simulink model "MVB1 - 副本"  (R2013b)
settings: Solver=ode3  StartTime=0.0  StopTime=6e-5  RelTol=1e-3
libraries: simulink x4
settings Model: Creator=qiji  LastModifiedBy=qiji
settings DataIOCC: SignalLoggingSaveFormat=ModelDataLogs
settings DebuggingCC: UnderspecifiedInitializationDetection=Simplified  MultiTaskDSMMsg=warning  MultiTaskCondExecSysMsg=none  SFUnusedDataAndEventsDiag=none
settings RTWCC: IncludeERTFirstTime=on
settings GRTTargetCC: CodeReplacementLibrary=None  CPPClassGenCompliant=on

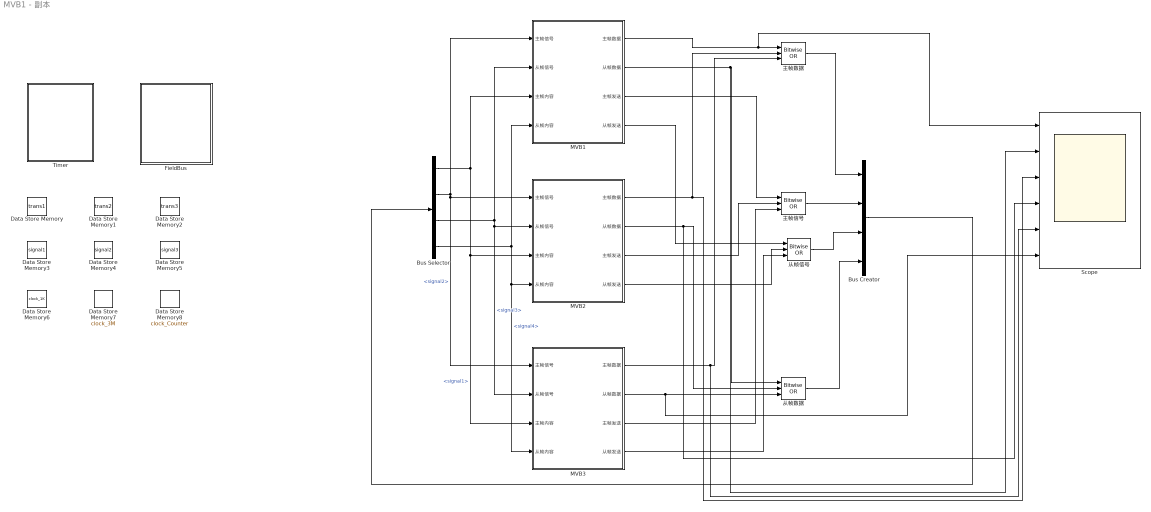
== system MVB1 - 副本 ==
  Bus Creator : BusCreator
  Bus Selector : BusSelector  OutputSignals=signal1,signal2,signal3,signal4
  Data Store Memory : DataStoreMemory  DataStoreName=trans1  ReadBeforeWriteMsg=warning  WriteAfterWriteMsg=warning  WriteAfterReadMsg=warning  OutDataTypeStr=boolean
  Data Store Memory1 : DataStoreMemory  DataStoreName=trans2  ReadBeforeWriteMsg=warning  WriteAfterWriteMsg=warning  WriteAfterReadMsg=warning  OutDataTypeStr=boolean
  Data Store Memory2 : DataStoreMemory  DataStoreName=trans3  ReadBeforeWriteMsg=warning  WriteAfterWriteMsg=warning  WriteAfterReadMsg=warning  OutDataTypeStr=boolean
  Data Store Memory3 : DataStoreMemory  DataStoreName=signal1  ReadBeforeWriteMsg=warning  WriteAfterWriteMsg=warning  WriteAfterReadMsg=warning  OutDataTypeStr=boolean
  Data Store Memory4 : DataStoreMemory  DataStoreName=signal2  ReadBeforeWriteMsg=warning  WriteAfterWriteMsg=warning  WriteAfterReadMsg=warning  OutDataTypeStr=boolean
  Data Store Memory5 : DataStoreMemory  DataStoreName=signal3  ReadBeforeWriteMsg=warning  WriteAfterWriteMsg=warning  WriteAfterReadMsg=warning  OutDataTypeStr=boolean
  Data Store Memory6 : DataStoreMemory  DataStoreName=clock_1K  ReadBeforeWriteMsg=warning  WriteAfterWriteMsg=warning  WriteAfterReadMsg=warning  OutDataTypeStr=boolean
  Data Store Memory7 : DataStoreMemory  DataStoreName=clock_3M  ReadBeforeWriteMsg=warning  WriteAfterWriteMsg=warning  WriteAfterReadMsg=warning  OutDataTypeStr=boolean
  Data Store Memory8 : DataStoreMemory  DataStoreName=clock_Counter  ReadBeforeWriteMsg=warning  WriteAfterWriteMsg=warning  WriteAfterReadMsg=warning  OutDataTypeStr=uint32
  FieldBus : Subsystem
  MVB1 : Subsystem
  MVB2 : Subsystem
  MVB3 : Subsystem
  Scope : Scope  NumInputPorts=6
      settings: YMin=0~0~0~0~0~0  YMax=3.5e+09~3e+09~3.5e+09~3e+09~3.5e+09~3e+09
  Timer : Subsystem
  主帧信号 : simulink/Logic and Bit Operations/Bitwise Operator  logicop=OR  UseBitMask=off  NumInputPorts=3  BitMask=bin2dec('11011001')  BitMaskRealWorld=Stored Integer
  主帧数据 : simulink/Logic and Bit Operations/Bitwise Operator  logicop=OR  UseBitMask=off  NumInputPorts=3  BitMask=bin2dec('11011001')  BitMaskRealWorld=Stored Integer
  从帧信号 : simulink/Logic and Bit Operations/Bitwise Operator  logicop=OR  UseBitMask=off  NumInputPorts=3  BitMask=bin2dec('11011001')  BitMaskRealWorld=Stored Integer
  从帧数据 : simulink/Logic and Bit Operations/Bitwise Operator  logicop=OR  UseBitMask=off  NumInputPorts=3  BitMask=bin2dec('11011001')  BitMaskRealWorld=Stored Integer
  wires:
  MVB1/1(主帧数据) -> Scope/1, 主帧数据/1
  MVB2/1(主帧数据) -> Scope/3, 主帧数据/2
  MVB3/1(主帧数据) -> Scope/5, 主帧数据/3
  MVB1/2(从帧数据) -> Scope/2, 从帧数据/1
  MVB2/2(从帧数据) -> 从帧数据/2, Scope/4
  MVB3/2(从帧数据) -> Scope/6, 从帧数据/3
  MVB1/3(主帧发送) -> 主帧信号/1
  MVB2/3(主帧发送) -> 主帧信号/2
  MVB3/3(主帧发送) -> 主帧信号/3
  MVB1/4(从帧发送) -> 从帧信号/1
  MVB2/4(从帧发送) -> 从帧信号/2
  MVB3/4(从帧发送) -> 从帧信号/3
  主帧数据/1 -> Bus Creator/1
  主帧信号/1 -> Bus Creator/2
  从帧信号/1 -> Bus Creator/3
  从帧数据/1 -> Bus Creator/4
  Bus Creator/1 -> Bus Selector/1
  Bus Selector/1 -> MVB2/3(主帧内容), MVB3/3(主帧内容), MVB1/3(主帧内容)  "<signal1>"
  Bus Selector/2 -> MVB3/1(主帧信号), MVB2/1(主帧信号), MVB1/1(主帧信号)  "<signal2>"
  Bus Selector/3 -> MVB3/2(从帧信号), MVB2/2(从帧信号), MVB1/2(从帧信号)  "<signal3>"
  Bus Selector/4 -> MVB3/4(从帧内容), MVB2/4(从帧内容), MVB1/4(从帧内容)  "<signal4>"

== system MVB1 - 副本/FieldBus ==
  FIELDBUS : Stateflow chart  TreatAsAtomicUnit=on

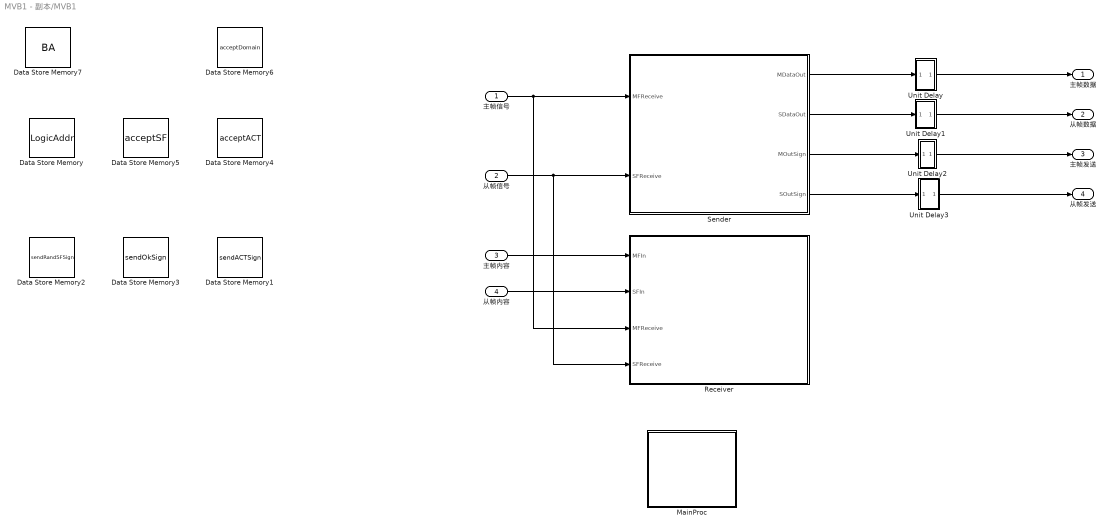
== system MVB1 - 副本/MVB1 ==
  主帧信号 : Inport
  从帧信号 : Inport  Port=2
  主帧内容 : Inport  Port=3
  从帧内容 : Inport  Port=4
  Data Store Memory : DataStoreMemory  DataStoreName=LogicAddr  ReadBeforeWriteMsg=warning  WriteAfterWriteMsg=warning  WriteAfterReadMsg=warning  InitialValue=1  OutDataTypeStr=uint32
  Data Store Memory1 : DataStoreMemory  DataStoreName=sendACTSign  ReadBeforeWriteMsg=warning  WriteAfterWriteMsg=warning  WriteAfterReadMsg=warning  OutDataTypeStr=boolean
  Data Store Memory2 : DataStoreMemory  DataStoreName=sendRandSFSign  ReadBeforeWriteMsg=warning  WriteAfterWriteMsg=warning  WriteAfterReadMsg=warning  OutDataTypeStr=boolean
  Data Store Memory3 : DataStoreMemory  DataStoreName=sendOkSign  ReadBeforeWriteMsg=warning  WriteAfterWriteMsg=warning  WriteAfterReadMsg=warning  OutDataTypeStr=boolean
  Data Store Memory4 : DataStoreMemory  DataStoreName=acceptACT  ReadBeforeWriteMsg=warning  WriteAfterWriteMsg=warning  WriteAfterReadMsg=warning  InitialValue=false  OutDataTypeStr=boolean
  Data Store Memory5 : DataStoreMemory  DataStoreName=acceptSF  ReadBeforeWriteMsg=warning  WriteAfterWriteMsg=warning  WriteAfterReadMsg=warning  InitialValue=false  OutDataTypeStr=boolean
  Data Store Memory6 : DataStoreMemory  DataStoreName=acceptDomain  ReadBeforeWriteMsg=warning  WriteAfterWriteMsg=warning  WriteAfterReadMsg=warning  InitialValue=false  OutDataTypeStr=boolean
  Data Store Memory7 : DataStoreMemory  DataStoreName=BA  ReadBeforeWriteMsg=warning  WriteAfterWriteMsg=warning  WriteAfterReadMsg=warning  InitialValue=true  OutDataTypeStr=boolean
  MainProc : Stateflow chart  TreatAsAtomicUnit=on
  Receiver : Stateflow chart  TreatAsAtomicUnit=on
  Sender : Stateflow chart  TreatAsAtomicUnit=on
  Unit Delay : Subsystem
  Unit Delay1 : Subsystem
  Unit Delay2 : Subsystem
  Unit Delay3 : Subsystem
  主帧数据 : Outport
  从帧数据 : Outport  Port=2
  主帧发送 : Outport  Port=3
  从帧发送 : Outport  Port=4
  wires:
  Sender/1(MDataOut) -> Unit Delay/1(In1)
  Sender/2(SDataOut) -> Unit Delay1/1(In1)
  Sender/3(MOutSign) -> Unit Delay2/1(In1)
  Sender/4(SOutSign) -> Unit Delay3/1(In1)
  Unit Delay/1(Out1) -> 主帧数据/1
  Unit Delay1/1(Out1) -> 从帧数据/1
  Unit Delay2/1(Out1) -> 主帧发送/1
  Unit Delay3/1(Out1) -> 从帧发送/1
  主帧信号/1 -> Receiver/3(MFReceive), Sender/1(MFReceive)
  从帧信号/1 -> Receiver/4(SFReceive), Sender/2(SFReceive)
  主帧内容/1 -> Receiver/1(MFIn)
  从帧内容/1 -> Receiver/2(SFIn)

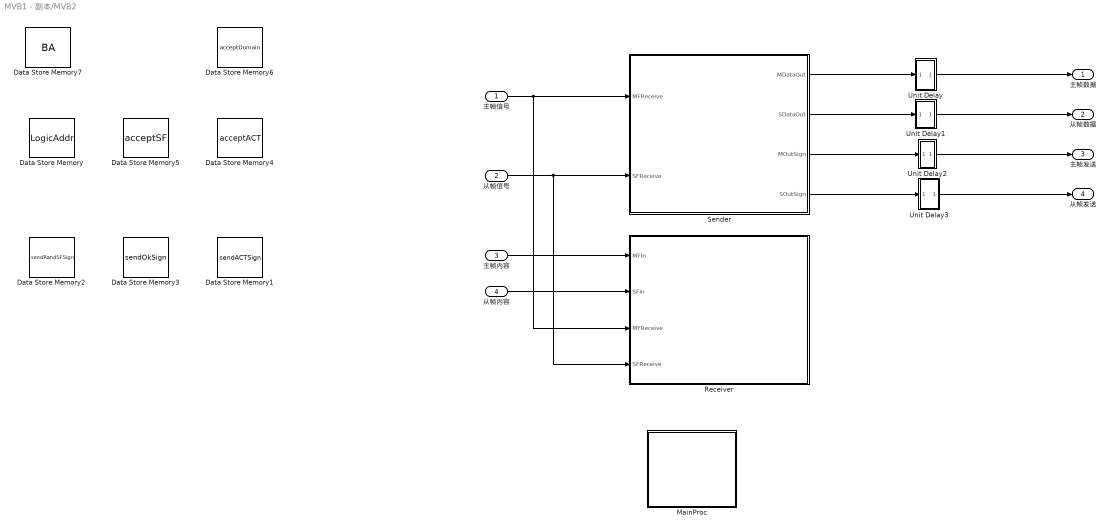
== system MVB1 - 副本/MVB2 ==
  主帧信号 : Inport
  从帧信号 : Inport  Port=2
  主帧内容 : Inport  Port=3
  从帧内容 : Inport  Port=4
  Data Store Memory : DataStoreMemory  DataStoreName=LogicAddr  ReadBeforeWriteMsg=warning  WriteAfterWriteMsg=warning  WriteAfterReadMsg=warning  InitialValue=2  OutDataTypeStr=uint32
  Data Store Memory1 : DataStoreMemory  DataStoreName=sendACTSign  ReadBeforeWriteMsg=warning  WriteAfterWriteMsg=warning  WriteAfterReadMsg=warning  OutDataTypeStr=boolean
  Data Store Memory2 : DataStoreMemory  DataStoreName=sendRandSFSign  ReadBeforeWriteMsg=warning  WriteAfterWriteMsg=warning  WriteAfterReadMsg=warning  OutDataTypeStr=boolean
  Data Store Memory3 : DataStoreMemory  DataStoreName=sendOkSign  ReadBeforeWriteMsg=warning  WriteAfterWriteMsg=warning  WriteAfterReadMsg=warning  OutDataTypeStr=boolean
  Data Store Memory4 : DataStoreMemory  DataStoreName=acceptACT  ReadBeforeWriteMsg=warning  WriteAfterWriteMsg=warning  WriteAfterReadMsg=warning  InitialValue=false  OutDataTypeStr=boolean
  Data Store Memory5 : DataStoreMemory  DataStoreName=acceptSF  ReadBeforeWriteMsg=warning  WriteAfterWriteMsg=warning  WriteAfterReadMsg=warning  InitialValue=false  OutDataTypeStr=boolean
  Data Store Memory6 : DataStoreMemory  DataStoreName=acceptDomain  ReadBeforeWriteMsg=warning  WriteAfterWriteMsg=warning  WriteAfterReadMsg=warning  InitialValue=false  OutDataTypeStr=boolean
  Data Store Memory7 : DataStoreMemory  DataStoreName=BA  ReadBeforeWriteMsg=warning  WriteAfterWriteMsg=warning  WriteAfterReadMsg=warning  InitialValue=true  OutDataTypeStr=boolean
  MainProc : Stateflow chart  TreatAsAtomicUnit=on
  Receiver : Stateflow chart  TreatAsAtomicUnit=on
  Sender : Stateflow chart  TreatAsAtomicUnit=on
  Unit Delay : Subsystem
  Unit Delay1 : Subsystem
  Unit Delay2 : Subsystem
  Unit Delay3 : Subsystem
  主帧数据 : Outport
  从帧数据 : Outport  Port=2
  主帧发送 : Outport  Port=3
  从帧发送 : Outport  Port=4
  wires:
  从帧内容/1 -> Receiver/2(SFIn)
  主帧内容/1 -> Receiver/1(MFIn)
  从帧信号/1 -> Sender/2(SFReceive), Receiver/4(SFReceive)
  主帧信号/1 -> Sender/1(MFReceive), Receiver/3(MFReceive)
  Unit Delay3/1(Out1) -> 从帧发送/1
  Unit Delay2/1(Out1) -> 主帧发送/1
  Unit Delay1/1(Out1) -> 从帧数据/1
  Unit Delay/1(Out1) -> 主帧数据/1
  Sender/4(SOutSign) -> Unit Delay3/1(In1)
  Sender/3(MOutSign) -> Unit Delay2/1(In1)
  Sender/2(SDataOut) -> Unit Delay1/1(In1)
  Sender/1(MDataOut) -> Unit Delay/1(In1)

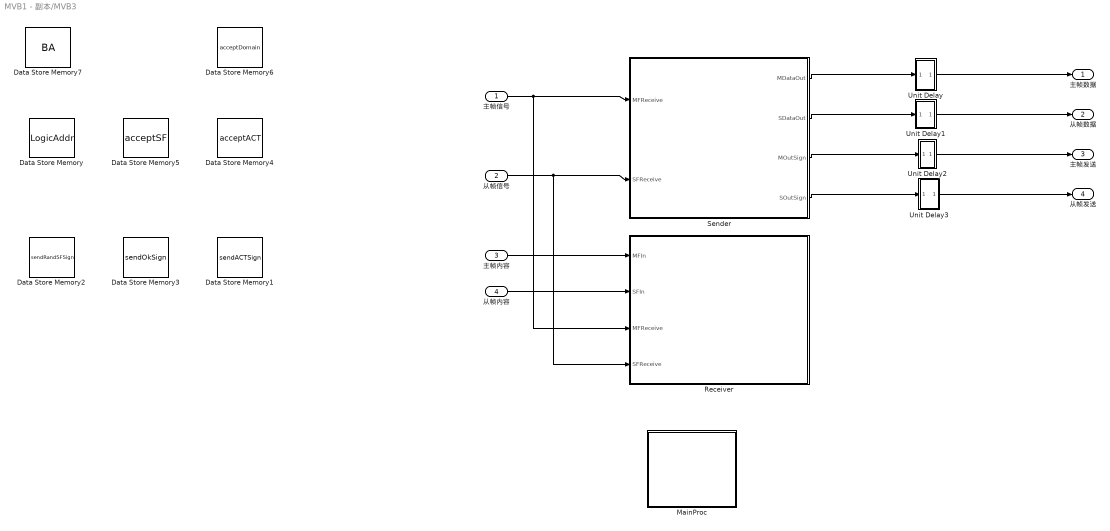
== system MVB1 - 副本/MVB3 ==
  主帧信号 : Inport
  从帧信号 : Inport  Port=2
  主帧内容 : Inport  Port=3
  从帧内容 : Inport  Port=4
  Data Store Memory : DataStoreMemory  DataStoreName=LogicAddr  ReadBeforeWriteMsg=warning  WriteAfterWriteMsg=warning  WriteAfterReadMsg=warning  InitialValue=3  OutDataTypeStr=uint32
  Data Store Memory1 : DataStoreMemory  DataStoreName=sendACTSign  ReadBeforeWriteMsg=warning  WriteAfterWriteMsg=warning  WriteAfterReadMsg=warning  OutDataTypeStr=boolean
  Data Store Memory2 : DataStoreMemory  DataStoreName=sendRandSFSign  ReadBeforeWriteMsg=warning  WriteAfterWriteMsg=warning  WriteAfterReadMsg=warning  OutDataTypeStr=boolean
  Data Store Memory3 : DataStoreMemory  DataStoreName=sendOkSign  ReadBeforeWriteMsg=warning  WriteAfterWriteMsg=warning  WriteAfterReadMsg=warning  OutDataTypeStr=boolean
  Data Store Memory4 : DataStoreMemory  DataStoreName=acceptACT  ReadBeforeWriteMsg=warning  WriteAfterWriteMsg=warning  WriteAfterReadMsg=warning  InitialValue=false  OutDataTypeStr=boolean
  Data Store Memory5 : DataStoreMemory  DataStoreName=acceptSF  ReadBeforeWriteMsg=warning  WriteAfterWriteMsg=warning  WriteAfterReadMsg=warning  InitialValue=false  OutDataTypeStr=boolean
  Data Store Memory6 : DataStoreMemory  DataStoreName=acceptDomain  ReadBeforeWriteMsg=warning  WriteAfterWriteMsg=warning  WriteAfterReadMsg=warning  InitialValue=false  OutDataTypeStr=boolean
  Data Store Memory7 : DataStoreMemory  DataStoreName=BA  ReadBeforeWriteMsg=warning  WriteAfterWriteMsg=warning  WriteAfterReadMsg=warning  InitialValue=true  OutDataTypeStr=boolean
  MainProc : Stateflow chart  TreatAsAtomicUnit=on
  Receiver : Stateflow chart  TreatAsAtomicUnit=on
  Sender : Stateflow chart  TreatAsAtomicUnit=on
  Unit Delay : Subsystem
  Unit Delay1 : Subsystem
  Unit Delay2 : Subsystem
  Unit Delay3 : Subsystem
  主帧数据 : Outport
  从帧数据 : Outport  Port=2
  主帧发送 : Outport  Port=3
  从帧发送 : Outport  Port=4
  wires:
  Sender/1(MDataOut) -> Unit Delay/1(In1)
  Sender/2(SDataOut) -> Unit Delay1/1(In1)
  Sender/3(MOutSign) -> Unit Delay2/1(In1)
  Sender/4(SOutSign) -> Unit Delay3/1(In1)
  Unit Delay/1(Out1) -> 主帧数据/1
  Unit Delay1/1(Out1) -> 从帧数据/1
  Unit Delay2/1(Out1) -> 主帧发送/1
  Unit Delay3/1(Out1) -> 从帧发送/1
  主帧信号/1 -> Receiver/3(MFReceive), Sender/1(MFReceive)
  从帧信号/1 -> Receiver/4(SFReceive), Sender/2(SFReceive)
  主帧内容/1 -> Receiver/1(MFIn)
  从帧内容/1 -> Receiver/2(SFIn)

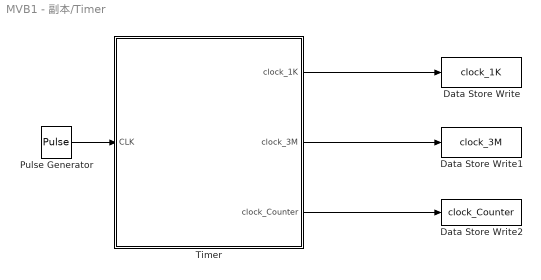
== system MVB1 - 副本/Timer ==
  Data Store Write : DataStoreWrite  DataStoreName=clock_1K
  Data Store Write1 : DataStoreWrite  DataStoreName=clock_3M
  Data Store Write2 : DataStoreWrite  DataStoreName=clock_Counter
  Pulse Generator : DiscretePulseGenerator  PulseType=Time based  Period=4.1666666667e-8  PulseWidth=50
  Timer : Stateflow chart  TreatAsAtomicUnit=on
  wires:
  Pulse Generator/1 -> Timer/1(CLK)
  Timer/3(clock_Counter) -> Data Store Write2/1
  Timer/2(clock_3M) -> Data Store Write1/1
  Timer/1(clock_1K) -> Data Store Write/1

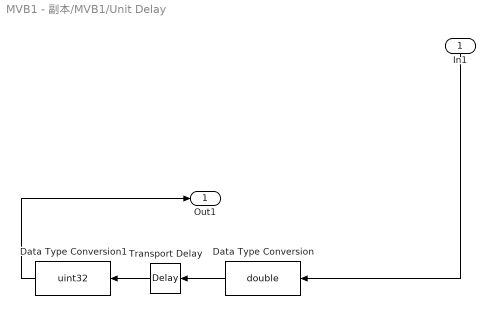
== system MVB1 - 副本/MVB1/Unit Delay ==
  In1 : Inport
  Data Type Conversion : DataTypeConversion  OutDataTypeStr=double
  Data Type Conversion1 : DataTypeConversion  OutDataTypeStr=uint32
  Transport Delay : TransportDelay  DelayTime=1e-7
  Out1 : Outport
  wires:
  In1/1 -> Data Type Conversion/1
  Data Type Conversion/1 -> Transport Delay/1
  Transport Delay/1 -> Data Type Conversion1/1
  Data Type Conversion1/1 -> Out1/1

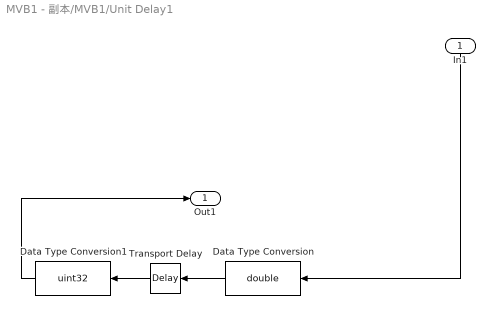
== system MVB1 - 副本/MVB1/Unit Delay1 ==
  In1 : Inport
  Data Type Conversion : DataTypeConversion  OutDataTypeStr=double
  Data Type Conversion1 : DataTypeConversion  OutDataTypeStr=uint32
  Transport Delay : TransportDelay  DelayTime=1e-7
  Out1 : Outport
  wires:
  In1/1 -> Data Type Conversion/1
  Data Type Conversion/1 -> Transport Delay/1
  Transport Delay/1 -> Data Type Conversion1/1
  Data Type Conversion1/1 -> Out1/1

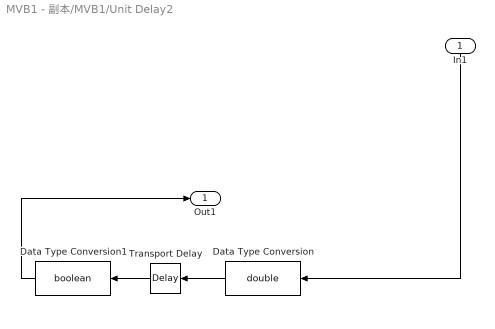
== system MVB1 - 副本/MVB1/Unit Delay2 ==
  In1 : Inport
  Data Type Conversion : DataTypeConversion  OutDataTypeStr=double
  Data Type Conversion1 : DataTypeConversion  OutDataTypeStr=boolean
  Transport Delay : TransportDelay  DelayTime=1e-7
  Out1 : Outport
  wires:
  In1/1 -> Data Type Conversion/1
  Data Type Conversion/1 -> Transport Delay/1
  Transport Delay/1 -> Data Type Conversion1/1
  Data Type Conversion1/1 -> Out1/1

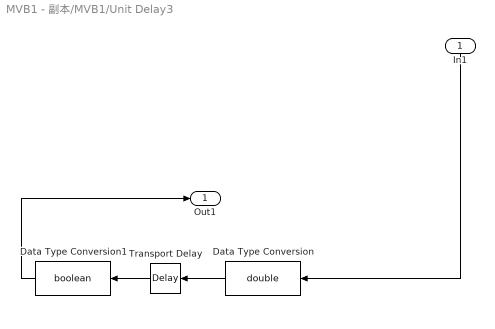
== system MVB1 - 副本/MVB1/Unit Delay3 ==
  In1 : Inport
  Data Type Conversion : DataTypeConversion  OutDataTypeStr=double
  Data Type Conversion1 : DataTypeConversion  OutDataTypeStr=boolean
  Transport Delay : TransportDelay  DelayTime=1e-7
  Out1 : Outport
  wires:
  In1/1 -> Data Type Conversion/1
  Data Type Conversion/1 -> Transport Delay/1
  Transport Delay/1 -> Data Type Conversion1/1
  Data Type Conversion1/1 -> Out1/1

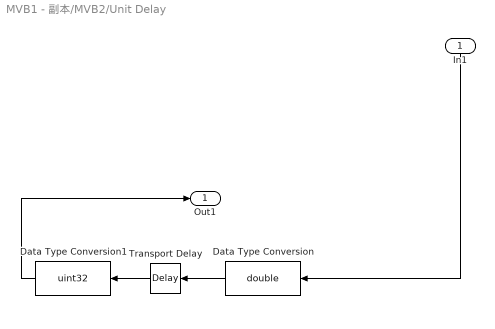
== system MVB1 - 副本/MVB2/Unit Delay ==
  In1 : Inport
  Data Type Conversion : DataTypeConversion  OutDataTypeStr=double
  Data Type Conversion1 : DataTypeConversion  OutDataTypeStr=uint32
  Transport Delay : TransportDelay  DelayTime=1e-7
  Out1 : Outport
  wires:
  Data Type Conversion1/1 -> Out1/1
  Transport Delay/1 -> Data Type Conversion1/1
  Data Type Conversion/1 -> Transport Delay/1
  In1/1 -> Data Type Conversion/1

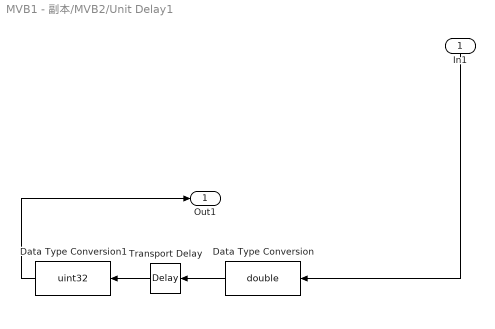
== system MVB1 - 副本/MVB2/Unit Delay1 ==
  In1 : Inport
  Data Type Conversion : DataTypeConversion  OutDataTypeStr=double
  Data Type Conversion1 : DataTypeConversion  OutDataTypeStr=uint32
  Transport Delay : TransportDelay  DelayTime=1e-7
  Out1 : Outport
  wires:
  Data Type Conversion1/1 -> Out1/1
  Transport Delay/1 -> Data Type Conversion1/1
  Data Type Conversion/1 -> Transport Delay/1
  In1/1 -> Data Type Conversion/1

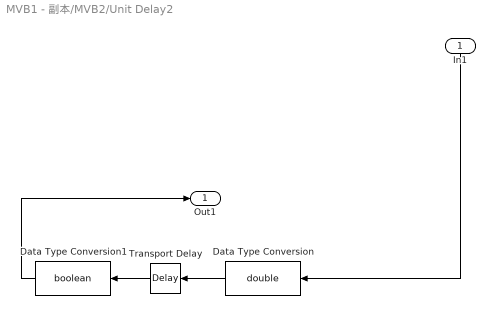
== system MVB1 - 副本/MVB2/Unit Delay2 ==
  In1 : Inport
  Data Type Conversion : DataTypeConversion  OutDataTypeStr=double
  Data Type Conversion1 : DataTypeConversion  OutDataTypeStr=boolean
  Transport Delay : TransportDelay  DelayTime=1e-7
  Out1 : Outport
  wires:
  Data Type Conversion1/1 -> Out1/1
  Transport Delay/1 -> Data Type Conversion1/1
  Data Type Conversion/1 -> Transport Delay/1
  In1/1 -> Data Type Conversion/1

== system MVB1 - 副本/MVB2/Unit Delay3 ==
  In1 : Inport
  Data Type Conversion : DataTypeConversion  OutDataTypeStr=double
  Data Type Conversion1 : DataTypeConversion  OutDataTypeStr=boolean
  Transport Delay : TransportDelay  DelayTime=1e-7
  Out1 : Outport
  wires:
  Data Type Conversion1/1 -> Out1/1
  Transport Delay/1 -> Data Type Conversion1/1
  Data Type Conversion/1 -> Transport Delay/1
  In1/1 -> Data Type Conversion/1

== system MVB1 - 副本/MVB3/Unit Delay ==
  In1 : Inport
  Data Type Conversion : DataTypeConversion  OutDataTypeStr=double
  Data Type Conversion1 : DataTypeConversion  OutDataTypeStr=uint32
  Transport Delay : TransportDelay  DelayTime=1e-7
  Out1 : Outport
  wires:
  In1/1 -> Data Type Conversion/1
  Data Type Conversion/1 -> Transport Delay/1
  Transport Delay/1 -> Data Type Conversion1/1
  Data Type Conversion1/1 -> Out1/1

== system MVB1 - 副本/MVB3/Unit Delay1 ==
  In1 : Inport
  Data Type Conversion : DataTypeConversion  OutDataTypeStr=double
  Data Type Conversion1 : DataTypeConversion  OutDataTypeStr=uint32
  Transport Delay : TransportDelay  DelayTime=1e-7
  Out1 : Outport
  wires:
  In1/1 -> Data Type Conversion/1
  Data Type Conversion/1 -> Transport Delay/1
  Transport Delay/1 -> Data Type Conversion1/1
  Data Type Conversion1/1 -> Out1/1

== system MVB1 - 副本/MVB3/Unit Delay2 ==
  In1 : Inport
  Data Type Conversion : DataTypeConversion  OutDataTypeStr=double
  Data Type Conversion1 : DataTypeConversion  OutDataTypeStr=boolean
  Transport Delay : TransportDelay  DelayTime=1e-7
  Out1 : Outport
  wires:
  In1/1 -> Data Type Conversion/1
  Data Type Conversion/1 -> Transport Delay/1
  Transport Delay/1 -> Data Type Conversion1/1
  Data Type Conversion1/1 -> Out1/1

== system MVB1 - 副本/MVB3/Unit Delay3 ==
  In1 : Inport
  Data Type Conversion : DataTypeConversion  OutDataTypeStr=double
  Data Type Conversion1 : DataTypeConversion  OutDataTypeStr=boolean
  Transport Delay : TransportDelay  DelayTime=1e-7
  Out1 : Outport
  wires:
  In1/1 -> Data Type Conversion/1
  Data Type Conversion/1 -> Transport Delay/1
  Transport Delay/1 -> Data Type Conversion1/1
  Data Type Conversion1/1 -> Out1/1

== stateflow chart MVB1 - 副本/FieldBus/FIELDBUS ==
  state IDLE
  state busy
  state space
  state turnFalse [function]
    (default) -> (junction 45) : {
        | trans1 = false;
        | trans2 = false;
        | trans3 = false;
        | }
  state r = pull(a, b, c) [function]
    (default) -> (junction 17)
    (junction 17) -> (junction 19) [order 1] : [a==true]{trans1=true; r=1;}
    (junction 17) -> (junction 21) [order 2]
    (junction 21) -> (junction 22) [order 1] : [b==true]{trans2=true; r=1;}
    (junction 21) -> (junction 24) [order 2]
    (junction 24) -> (junction 23) : [c==true]{trans3=true;r=1}
  state init [function]
    (default) -> (junction 40) : {
        | trans1 = false;
        | trans2 = false;
        | trans3 = false;
        | }
  IDLE -> busy : [pull(signal1, signal2, signal3)]
  (default) -> IDLE
  busy -> space : {t = clock_Counter}
  space -> IDLE : [clock_Counter - t > 488]{turnFalse()}
  data: r function_output double; a function_input double; b function_input double; c function_input double; t local uint32; clock_Counter data_store_memory; trans1 data_store_memory; trans2 data_store_memory; trans3 data_store_memory; signal1 data_store_memory; signal2 data_store_memory; signal3 data_store_memory

== stateflow chart MVB1 - 副本/Timer/Timer ==
  state ClockManager
    note: 时钟模块
    state initTimer [function]
      (default) -> (junction 13) : {
          | clock1K_Counter = uint32(0);
          | clock3M_Counter = uint32(0);
          | clock_Counter = uint32(0);
          | clock_1K = true;
          | clock_3M = true;
          | }
    state ClockStart
    state Devider
      state startDevider
      startDevider -> (junction 7) : [CLK==1]
      (junction 7) -> (junction 8) [order 1] : [clock1K_Counter == 24000]
          | {
          | clock_1K = ~clock_1K;
          | clock1K_Counter = uint32(0);
          | }
      (junction 7) -> (junction 10) [order 2]
      (junction 8) -> (junction 10)
      (default) -> startDevider
      (junction 10) -> (junction 11) [order 1] : [clock3M_Counter == 50]
          | {
          | clock_3M = 1 - clock_3M;
          | clock3M_Counter = uint32(0);
          | }
      (junction 10) -> (junction 15) [order 2]
      (junction 15) -> startDevider : {
          | clock3M_Counter = clock3M_Counter + 1;
          | clock1K_Counter = clock1K_Counter + 1;
          | clock_Counter = clock_Counter + 1;
          | }
      (junction 11) -> (junction 15)
    (default) -> ClockStart
    ClockStart -> Devider : {
        | initTimer()
        | }
  data: clock1K_Counter local uint32; clock3M_Counter local uint32; clock_1K output boolean; clock_3M output boolean; clock_Counter output uint32; CLK input double

== stateflow chart MVB1 - 副本/MVB1/Sender ==
  state init [function]
    note: 请求随机从帧
        | 请求随机从帧
        | 请求2号的信息
        | 请求转移到2号
    note: SFT(1)代表随机的从帧
        | SFT(2)代表回复接受主权
        | SFT(3)代表回复设备LAT和BA
    (default) -> (junction 100) : {
        | BA = true;
        | MFIndex = 1;
        | isMaster = true;
        | SendSignal = false;
        | MFT(1) = getMF(0, 2);
        | MFT(2) = getMF(0, 3);
        | MFT(3) = getMF(15, 2);
        | MFT(4) = getMF(8, 2);
        | MFT(5) = 1;
        | SFT(1) = getSF(777);
        | SFT(2) = getSF(32768);
        | SFT(3) = getSF(16512);
        | clock_3M_shang = false;
        | sendRandSFSign = false;
        | sendACTSign = false;
        | sendRandSFSign = false;
        | }
  state SFSender [parallel]
    settings: executionOrder=1
    note: send**Signd的置位在接收到了请求数据的主帧后置位
    state sender [parallel]
      settings: executionOrder=1
      state wait
      state sendInfo
      state sendRandomSF
      state sendOK
      state transmission
        entry:
        SDataOut = SFT(SFIndex);
        SOutSign = true;
      (default) -> SFSender.sender.wait
      SFSender.sender.wait -> sendRandomSF [order 1] : [sendRandSFSign == true]
      SFSender.sender.wait -> sendOK [order 2] : [sendOkSign == true]
          | {
          | isMaster = true;
          | }
      SFSender.sender.wait -> sendInfo [order 3] : [sendACTSign == true]
      sendInfo -> SFSender.sender.transmission : {SFIndex = 3;
          | sendACTSign = false;}
      sendRandomSF -> SFSender.sender.transmission : {SFIndex = 1;
          | sendRandSFSign = false;}
      sendOK -> SFSender.sender.transmission : {SFIndex = 2;
          | sendOkSign = false;
          | init();
          | BA = true;
          | }
      SFSender.sender.transmission -> SFSender.sender : exit(SendHolder.hold)
          | {SDataOut = uint32(0);
          | SOutSign = false;
          | }
    state SendHolder [parallel]
      settings: executionOrder=2
      state end
      state hold
      note: 数据的发送需要持续42.7us
      end -> hold : enter(sender.transmission)
          | {
          | t1 = clock_Counter;
          | }
      (default) -> end
      hold -> end : [clock_Counter - t1 > 4.27]
  state MFSender [parallel]
    settings: executionOrder=2
    state sender [parallel]
      settings: executionOrder=1
      state sleep
      state wait
        entry:
        signal1 = true
      state transmission
        entry:
        signal1 = false;
        MDataOut = MFT(MFIndex);
        MOutSign = true;
        [acceptSF, acceptACT, acceptDomain] = setAcceptSignal(MDataOut);
      (default) -> sleep : {
          | init();
          | }
      sleep -> MFSender.sender.wait : [BA==true && clock_3M ~= clock_3M_shang]
          | {
          | clock_3M_shang = clock_3M;
          | }
      MFSender.sender.transmission -> sleep : exit(buffer.full)
          | {
          | MDataOut = uint32(0);
          | MOutSign = false;
          | MFIndex = MFIndex + 1;
          | }
      MFSender.sender.wait -> MFSender.sender.transmission : [trans1 == true]
    state buffer [parallel]
      settings: executionOrder=2
      note: 输出要保持42.7us
      state full
      state empty
      (default) -> empty
      full -> empty : [clock_Counter - t2 > 4.27]
      empty -> full : [enter(sender.transmission)]
          | {
          | t2 = clock_Counter;
          | }
  (default) -> MFSender
  data: f_code function_input; addr function_input; r function_output; addr function_input; r function_output; SFIndex local double; t1 local uint32; dataIn function_input uint32; SF function_output boolean; ACT function_output; Domain function_output; t2 local uint32; MFReceive input boolean; MDataOut output uint32; clock_3M data_store_memory; clock_Counter data_store_memory; MFIndex local; MFT local uint32 size=5; trans1 data_store_memory; signal1 data_store_memory; SFReceive input boolean; sendOkSign data_store_memory; sendRandSFSign data_store_memory; sendACTSign data_store_memory; SFT local uint32 size=3; SDataOut output uint32; MOutSign output boolean; SOutSign output boolean; isMaster local boolean; acceptSF data_store_memory; BA data_store_memory; clock_3M_shang local boolean; acceptACT data_store_memory; acceptDomain data_store_memory
  function r = getMF(f_code, addr):
    | function r = getMF(f_code, addr)
    | r = 3340042240;
    | r = r + bitshift(uint32(f_code), 12);
    | r = r + addr;
  function r = getSF(addr):
    | function r = getSF(addr)
    | r = 2833448960;
    | r = r + addr;
  function judgeMaster:
    | function judgeMaster
    | % 如果
    | if isMaster == true && SFIndex == 2
    |     isMaster = false;
    | end
  function [SF, ACT, Domain] = setAcceptSignal(dataIn):
    | function [SF, ACT, Domain] = setAcceptSignal(dataIn)
    | % 右移12位 仅保留帧头和fcode
    | dataInExAddr = bitshift(uint32(dataIn), -12);
    | % 先右移16位再左移4位 仅仅保留帧头
    | dataInStart = bitshift(bitshift(uint32(dataIn), -16), 4);
    | % 相减得到fcode
    | fcode = double(dataInExAddr - dataInStart);
    | SF = false;
    | Domain = false;
    | ACT = false;
    | if fcode == 0
    |     SF = true;
    | elseif fcode == 15
    |     ACT = true;
    | else
    |     Domain = true;
    | end

== stateflow chart MVB1 - 副本/MVB1/Receiver ==
  state wait
  note: acceptSF, acceptACT, acceptDomain在发送完主帧以后，根据主帧的类型进行相应的置位
      | 收到fcode为8的从帧之后，说明目标设备已经返回了OK，这时应该将ismaster设为1
  state judge4SF
  state judgeAddr
  note: 期待目标设备返回OK
  state wait4SF
  state wait4ACT
  state wait4Domain
  state MFReceive
  state MFcode0
  state MFcode8
  state MFcode15
  state STrans
  state MTrans
  (default) -> wait : {
      | t = clock_Counter;
      | }
  (junction 96) -> wait
  wait -> judge4SF [order 2] : [SFReceive== true]
      | {
      | t = 0;
      | }
  MTrans -> wait : [sendRandSFSign == false && sendOkSign == false && sendACTSign == false]
      | {
      | t = clock_Counter;
      | }
  judgeAddr -> wait [order 2]
  wait -> judgeAddr [order 1] : [MFReceive==true]
      | {
      | fcodeIn = uint8(getFCode(MFIn));
      | addrIn = uint16(getAddr(MFIn));
      | t = 0;
      | }
  judge4SF -> wait4Domain [order 3] : [acceptDomain == true]
  judge4SF -> (junction 96) [order 4]
  judge4SF -> wait4SF [order 1] : [acceptSF == true]
  STrans -> (junction 96) : [SFReceive == false]
  judge4SF -> wait4ACT [order 2] : [acceptACT == true]
  judgeAddr -> MFReceive [order 1] : [addrIn == LogicAddr]
  wait4SF -> STrans : {
      | acceptSF = false;
      | }
  wait4ACT -> STrans : [getbit(SFIn, 8)]
      | {
      | acceptACT = false;
      | }
  wait4Domain -> STrans : [getbit(SFIn, 16) == 1]
      | {
      | acceptDomain = false;
      | BA = false;
      | }
  MFReceive -> MFcode0 [order 2] : [fcodeIn == 0 && MFReceive == false ]
  MFReceive -> MFcode8 [order 3] : [fcodeIn == 8 && MFReceive == false]
  MFReceive -> MFcode15 [order 1] : [fcodeIn == 15 && MFReceive == false]
  MFcode0 -> MTrans : {sendRandSFSign = true}
  MFcode8 -> MTrans : {sendOkSign = true}
  MFcode15 -> MTrans : {sendACTSign = true}
  data: dataIn function_input double; r function_output double; dataIn function_input double; r function_output double; dataIn function_input uint32; num function_input uint32; r function_output uint32; MFIn input uint32; SFIn input uint32; t local uint32; clock_Counter data_store_memory; clock_3M data_store_memory; MFReceive input boolean; SFReceive input boolean; fcodeIn local uint8; addrIn local uint16; trans1 data_store_memory; LogicAddr data_store_memory; sendRandSFSign data_store_memory; sendOkSign data_store_memory; sendACTSign data_store_memory; acceptSF data_store_memory; acceptDomain data_store_memory; acceptACT data_store_memory; BA data_store_memory
  function r = getFCode(dataIn):
    | function r = getFCode(dataIn)
    | % 右移12位 仅保留帧头和fcode
    | dataInExAddr = bitshift(uint32(dataIn), -12);
    | % 先右移16位再左移4位 仅仅保留帧头
    | dataInStart = bitshift(bitshift(uint32(dataIn), -16), 4);
    | % 相减得到fcode
    | r = double(dataInExAddr - dataInStart);
  function r = getAddr(dataIn):
    | function r = getAddr(dataIn)
    | % 把后12位也就是地址归零
    | dataInExAddr = bitshift(bitshift(uint32(dataIn), -12), 12);
    | % 相减获取地址
    | r = double(dataIn - dataInExAddr);
  function r = getbit(dataIn, num):
    | function r = getbit(dataIn, num)
    | r = bitget(uint32(dataIn), num);

== stateflow chart MVB1 - 副本/MVB1/MainProc ==
  state StandbyEquip
  state MainEquip
  note: 等待其他设备返回ACT
  state wait4ACT
  note: 等待其他设备返回OK，receiver在接收到OK以后立马放弃主权
  state TempEquip
  (default) -> StandbyEquip
  TempEquip -> StandbyEquip : [BA == false]
  StandbyEquip -> MainEquip : [BA == true && ACT == true]
  MainEquip -> wait4ACT : [acceptACT == true]
      | {
      | t = clock_Counter;
      | }
  wait4ACT -> TempEquip : [acceptDomain == true]
      | {
      | t = clock_Counter;
      | }
  data: BA data_store_memory; ACT local boolean =true; acceptACT data_store_memory; acceptDomain data_store_memory; t local uint32; clock_Counter data_store_memory

== stateflow chart MVB1 - 副本/MVB2/MainProc ==
  state StandbyEquip
  state MainEquip
  note: 等待其他设备返回ACT
  state wait4ACT
  note: 等待其他设备返回OK，receiver在接收到OK以后立马放弃主权
  state TempEquip
  (default) -> StandbyEquip
  TempEquip -> StandbyEquip [order 2] : [BA == false]
  wait4ACT -> StandbyEquip [order 3]
  StandbyEquip -> MainEquip : [BA == true && ACT == true]
  MainEquip -> wait4ACT : [acceptACT == true]
      | {
      | t = clock_Counter;
      | }
  (junction 16) -> wait4ACT
  wait4ACT -> (junction 16) [order 1] : [clock_Counter - t < 9.6]
  wait4ACT -> TempEquip [order 2] : [acceptDomain == true]
      | {
      | t = clock_Counter;
      | }
  (junction 20) -> TempEquip
  TempEquip -> (junction 20) [order 1] : [clock_Counter - t < 9.6]
  data: BA data_store_memory; ACT local boolean =true; acceptACT data_store_memory; acceptDomain data_store_memory; t local uint32; clock_Counter data_store_memory

== stateflow chart MVB1 - 副本/MVB2/Receiver ==
  state wait
  note: acceptSF, acceptACT, acceptDomain在发送完主帧以后，根据主帧的类型进行相应的置位
      | 收到fcode为8的从帧之后，说明目标设备已经返回了OK，这时应该将ismaster设为1
  state judge4SF
  state judgeAddr
  note: 期待目标设备返回OK
  state wait4SF
  state wait4ACT
  state wait4Domain
  state MFReceive
  state MFcode0
  state MFcode8
  state MFcode15
  state STrans
  state MTrans
  (default) -> wait : {
      | t = clock_Counter;
      | }
  (junction 96) -> wait
  wait -> judge4SF [order 2] : [SFReceive== true]
      | {
      | t = 0;
      | }
  MTrans -> wait : [sendRandSFSign == false && sendOkSign == false && sendACTSign == false]
      | {
      | t = clock_Counter;
      | }
  judgeAddr -> wait [order 2]
  wait -> judgeAddr [order 1] : [MFReceive==true]
      | {
      | fcodeIn = uint8(getFCode(MFIn));
      | addrIn = uint16(getAddr(MFIn));
      | t = 0;
      | }
  judge4SF -> wait4Domain [order 3] : [acceptDomain == true]
  judge4SF -> (junction 96) [order 4]
  judge4SF -> wait4SF [order 1] : [acceptSF == true]
  STrans -> (junction 96) : [SFReceive == false]
  judge4SF -> wait4ACT [order 2] : [acceptACT == true]
  judgeAddr -> MFReceive [order 1] : [addrIn == LogicAddr]
  wait4SF -> STrans : {
      | acceptSF = false;
      | }
  wait4ACT -> STrans : [getbit(SFIn, 8)]
      | {
      | acceptACT = false;
      | }
  wait4Domain -> STrans : [getbit(SFIn, 16) == 1]
      | {
      | acceptDomain = false;
      | BA = false;
      | }
  MFReceive -> MFcode0 [order 2] : [fcodeIn == 0 && MFReceive == false ]
  MFReceive -> MFcode8 [order 3] : [fcodeIn == 8 && MFReceive == false]
  MFReceive -> MFcode15 [order 1] : [fcodeIn == 15 && MFReceive == false]
  MFcode0 -> MTrans : {sendRandSFSign = true}
  MFcode8 -> MTrans : {sendOkSign = true}
  MFcode15 -> MTrans : {sendACTSign = true}
  data: dataIn function_input double; r function_output double; dataIn function_input double; r function_output double; dataIn function_input uint32; num function_input uint32; r function_output uint32; MFIn input uint32; SFIn input uint32; t local uint32; clock_Counter data_store_memory; clock_3M data_store_memory; MFReceive input boolean; SFReceive input boolean; fcodeIn local uint8; addrIn local uint16; trans1 data_store_memory; LogicAddr data_store_memory; sendRandSFSign data_store_memory; sendOkSign data_store_memory; sendACTSign data_store_memory; acceptSF data_store_memory; acceptDomain data_store_memory; acceptACT data_store_memory; BA data_store_memory
  function r = getFCode(dataIn):
    | function r = getFCode(dataIn)
    | % 右移12位 仅保留帧头和fcode
    | dataInExAddr = bitshift(uint32(dataIn), -12);
    | % 先右移16位再左移4位 仅仅保留帧头
    | dataInStart = bitshift(bitshift(uint32(dataIn), -16), 4);
    | % 相减得到fcode
    | r = double(dataInExAddr - dataInStart);
  function r = getAddr(dataIn):
    | function r = getAddr(dataIn)
    | % 把后12位也就是地址归零
    | dataInExAddr = bitshift(bitshift(uint32(dataIn), -12), 12);
    | % 相减获取地址
    | r = double(dataIn - dataInExAddr);
  function r = getbit(dataIn, num):
    | function r = getbit(dataIn, num)
    | r = bitget(uint32(dataIn), num);

== stateflow chart MVB1 - 副本/MVB2/Sender ==
  state init [function]
    note: 请求随机从帧
        | 请求随机从帧
        | 请求2号的信息
        | 请求转移到2号
    note: SFT(1)代表随机的从帧
        | SFT(2)代表回复接受主权
        | SFT(3)代表回复设备LAT和BA
    (default) -> (junction 100) : {
        | BA = false;
        | MFIndex = 1;
        | isMaster = true;
        | SendSignal = false;
        | MFT(1) = getMF(0, 1);
        | MFT(2) = getMF(0, 3);
        | MFT(3) = getMF(15, 3);
        | MFT(4) = getMF(8, 3);
        | MFT(5) = 1;
        | SFT(1) = getSF(777);
        | SFT(2) = getSF(32768);
        | SFT(3) = getSF(16512);
        | clock_3M_shang = false;
        | sendRandSFSign = false;
        | sendACTSign = false;
        | sendOkSign = false;
        | }
  state SFSender [parallel]
    settings: executionOrder=1
    note: send**Signd的置位在接收到了请求数据的主帧后置位
    state sender [parallel]
      settings: executionOrder=1
      state wait
      state sendInfo
      state sendRandomSF
      state sendOK
      state transmission
        entry:
        SDataOut = SFT(SFIndex);
        SOutSign = true;
      (default) -> SFSender.sender.wait
      SFSender.sender.wait -> sendRandomSF [order 1] : [sendRandSFSign == true]
      SFSender.sender.wait -> sendOK [order 2] : [sendOkSign == true]
          | {
          | isMaster = true;
          | }
      SFSender.sender.wait -> sendInfo [order 3] : [sendACTSign == true]
      sendInfo -> SFSender.sender.transmission : {SFIndex = 3;
          | sendACTSign = false;}
      sendRandomSF -> SFSender.sender.transmission : {SFIndex = 1;
          | sendRandSFSign = false;}
      sendOK -> SFSender.sender.transmission : {SFIndex = 2;
          | sendOkSign = false;
          | init();
          | BA = true;
          | }
      SFSender.sender.transmission -> SFSender.sender : exit(SendHolder.hold)
          | {SDataOut = uint32(0);
          | SOutSign = false;
          | }
    state SendHolder [parallel]
      settings: executionOrder=2
      state end
      state hold
      note: 数据的发送需要持续42.7us
      end -> hold : enter(sender.transmission)
          | {
          | t1 = clock_Counter;
          | }
      (default) -> end
      hold -> end : [clock_Counter - t1 > 4.27]
  state MFSender [parallel]
    settings: executionOrder=2
    state sender [parallel]
      settings: executionOrder=1
      state sleep
      state wait
        entry:
        signal1 = true
      state transmission
        entry:
        signal1 = false;
        MDataOut = MFT(MFIndex);
        MOutSign = true;
        [acceptSF, acceptACT, acceptDomain] = setAcceptSignal(MDataOut);
      (default) -> sleep : {
          | init();
          | }
      sleep -> MFSender.sender.wait : [BA==true && clock_3M ~= clock_3M_shang]
          | {
          | clock_3M_shang = clock_3M;
          | }
      MFSender.sender.transmission -> sleep : exit(buffer.full)
          | {
          | MDataOut = uint32(0);
          | MOutSign = false;
          | MFIndex = MFIndex + 1;
          | }
      MFSender.sender.wait -> MFSender.sender.transmission : [trans1 == true]
    state buffer [parallel]
      settings: executionOrder=2
      note: 输出要保持42.7us
      state full
      state empty
      (default) -> empty
      full -> empty : [clock_Counter - t2 > 4.27]
      empty -> full : [enter(sender.transmission)]
          | {
          | t2 = clock_Counter;
          | }
  (default) -> MFSender
  data: f_code function_input; addr function_input; r function_output; addr function_input; r function_output; SFIndex local double; t1 local uint32; dataIn function_input uint32; SF function_output boolean; ACT function_output; Domain function_output; t2 local uint32; MFReceive input boolean; MDataOut output uint32; clock_3M data_store_memory; clock_Counter data_store_memory; MFIndex local; MFT local uint32 size=5; trans1 data_store_memory; signal1 data_store_memory; SFReceive input boolean; sendOkSign data_store_memory; sendRandSFSign data_store_memory; sendACTSign data_store_memory; SFT local uint32 size=3; SDataOut output uint32; MOutSign output boolean; SOutSign output boolean; isMaster local boolean; acceptSF data_store_memory; BA data_store_memory; clock_3M_shang local boolean; acceptACT data_store_memory; acceptDomain data_store_memory
  function r = getMF(f_code, addr):
    | function r = getMF(f_code, addr)
    | r = 3340042240;
    | r = r + bitshift(uint32(f_code), 12);
    | r = r + addr;
  function r = getSF(addr):
    | function r = getSF(addr)
    | r = 2833448960;
    | r = r + addr;
  function judgeMaster:
    | function judgeMaster
    | % 如果
    | if isMaster == true && SFIndex == 2
    |     isMaster = false;
    | end
  function [SF, ACT, Domain] = setAcceptSignal(dataIn):
    | function [SF, ACT, Domain] = setAcceptSignal(dataIn)
    | % 右移12位 仅保留帧头和fcode
    | dataInExAddr = bitshift(uint32(dataIn), -12);
    | % 先右移16位再左移4位 仅仅保留帧头
    | dataInStart = bitshift(bitshift(uint32(dataIn), -16), 4);
    | % 相减得到fcode
    | fcode = double(dataInExAddr - dataInStart);
    | SF = false;
    | Domain = false;
    | ACT = false;
    | if fcode == 0
    |     SF = true;
    | elseif fcode == 15
    |     ACT = true;
    | else
    |     Domain = true;
    | end

== stateflow chart MVB1 - 副本/MVB3/MainProc ==
  state StandbyEquip
  state MainEquip
  note: 等待其他设备返回ACT
  state wait4ACT
  note: 等待其他设备返回OK，receiver在接收到OK以后立马放弃主权
  state TempEquip
  (default) -> StandbyEquip
  TempEquip -> StandbyEquip [order 2] : [BA == false]
  wait4ACT -> StandbyEquip [order 3]
  StandbyEquip -> MainEquip : [BA == true && ACT == true]
  MainEquip -> wait4ACT : [acceptACT == true]
      | {
      | t = clock_Counter;
      | }
  (junction 16) -> wait4ACT
  wait4ACT -> (junction 16) [order 1] : [clock_Counter - t < 9.6]
  wait4ACT -> TempEquip [order 2] : [acceptDomain == true]
      | {
      | t = clock_Counter;
      | }
  (junction 20) -> TempEquip
  TempEquip -> (junction 20) [order 1] : [clock_Counter - t < 9.6]
  data: BA data_store_memory; ACT local boolean =true; acceptACT data_store_memory; acceptDomain data_store_memory; t local uint32; clock_Counter data_store_memory

== stateflow chart MVB1 - 副本/MVB3/Receiver ==
  state wait
  note: acceptSF, acceptACT, acceptDomain在发送完主帧以后，根据主帧的类型进行相应的置位
      | 收到fcode为8的从帧之后，说明目标设备已经返回了OK，这时应该将ismaster设为1
  state judge4SF
  state judgeAddr
  note: 期待目标设备返回OK
  state wait4SF
  state wait4ACT
  state wait4Domain
  state MFReceive
  state MFcode0
  state MFcode8
  state MFcode15
  state STrans
  state MTrans
  (default) -> wait : {
      | t = clock_Counter;
      | }
  (junction 96) -> wait
  wait -> judge4SF [order 2] : [SFReceive== true]
      | {
      | t = 0;
      | }
  MTrans -> wait : [sendRandSFSign == false && sendOkSign == false && sendACTSign == false]
      | {
      | t = clock_Counter;
      | }
  judgeAddr -> wait [order 2]
  wait -> judgeAddr [order 1] : [MFReceive==true]
      | {
      | fcodeIn = uint8(getFCode(MFIn));
      | addrIn = uint16(getAddr(MFIn));
      | t = 0;
      | }
  judge4SF -> wait4Domain [order 3] : [acceptDomain == true]
  judge4SF -> (junction 96) [order 4]
  judge4SF -> wait4SF [order 1] : [acceptSF == true]
  STrans -> (junction 96) : [SFReceive == false]
  judge4SF -> wait4ACT [order 2] : [acceptACT == true]
  judgeAddr -> MFReceive [order 1] : [addrIn == LogicAddr]
  wait4SF -> STrans : {
      | acceptSF = false;
      | }
  wait4ACT -> STrans : [getbit(SFIn, 8)]
      | {
      | acceptACT = false;
      | }
  wait4Domain -> STrans : [getbit(SFIn, 16) == 1]
      | {
      | acceptDomain = false;
      | BA = false;
      | }
  MFReceive -> MFcode0 [order 2] : [fcodeIn == 0 && MFReceive == false ]
  MFReceive -> MFcode8 [order 3] : [fcodeIn == 8 && MFReceive == false]
  MFReceive -> MFcode15 [order 1] : [fcodeIn == 15 && MFReceive == false]
  MFcode0 -> MTrans : {sendRandSFSign = true}
  MFcode8 -> MTrans : {sendOkSign = true}
  MFcode15 -> MTrans : {sendACTSign = true}
  data: dataIn function_input double; r function_output double; dataIn function_input double; r function_output double; dataIn function_input uint32; num function_input uint32; r function_output uint32; MFIn input uint32; SFIn input uint32; t local uint32; clock_Counter data_store_memory; clock_3M data_store_memory; MFReceive input boolean; SFReceive input boolean; fcodeIn local uint8; addrIn local uint16; trans1 data_store_memory; LogicAddr data_store_memory; sendRandSFSign data_store_memory; sendOkSign data_store_memory; sendACTSign data_store_memory; acceptSF data_store_memory; acceptDomain data_store_memory; acceptACT data_store_memory; BA data_store_memory
  function r = getFCode(dataIn):
    | function r = getFCode(dataIn)
    | % 右移12位 仅保留帧头和fcode
    | dataInExAddr = bitshift(uint32(dataIn), -12);
    | % 先右移16位再左移4位 仅仅保留帧头
    | dataInStart = bitshift(bitshift(uint32(dataIn), -16), 4);
    | % 相减得到fcode
    | r = double(dataInExAddr - dataInStart);
  function r = getAddr(dataIn):
    | function r = getAddr(dataIn)
    | % 把后12位也就是地址归零
    | dataInExAddr = bitshift(bitshift(uint32(dataIn), -12), 12);
    | % 相减获取地址
    | r = double(dataIn - dataInExAddr);
  function r = getbit(dataIn, num):
    | function r = getbit(dataIn, num)
    | r = bitget(uint32(dataIn), num);

== stateflow chart MVB1 - 副本/MVB3/Sender ==
  state init [function]
    note: 请求随机从帧
        | 请求随机从帧
        | 请求2号的信息
        | 请求转移到2号
    note: SFT(1)代表随机的从帧
        | SFT(2)代表回复接受主权
        | SFT(3)代表回复设备LAT和BA
    (default) -> (junction 100) : {
        | BA = false;
        | MFIndex = 1;
        | isMaster = true;
        | SendSignal = false;
        | MFT(1) = getMF(0, 1);
        | MFT(2) = getMF(0, 2);
        | MFT(3) = getMF(15, 1);
        | MFT(4) = getMF(8, 1);
        | MFT(5) = 1;
        | SFT(1) = getSF(777);
        | SFT(2) = getSF(32768);
        | SFT(3) = getSF(16512);
        | clock_3M_shang = false;
        | sendRandSFSign = false;
        | sendOkSign = false;
        | sendACTSign = false;
        | }
  state SFSender [parallel]
    settings: executionOrder=1
    note: send**Signd的置位在接收到了请求数据的主帧后置位
    state sender [parallel]
      settings: executionOrder=1
      state wait
      state sendInfo
      state sendRandomSF
      state sendOK
      state transmission
        entry:
        SDataOut = SFT(SFIndex);
        SOutSign = true;
      (default) -> SFSender.sender.wait
      SFSender.sender.wait -> sendRandomSF [order 1] : [sendRandSFSign == true]
      SFSender.sender.wait -> sendOK [order 2] : [sendOkSign == true]
          | {
          | isMaster = true;
          | }
      SFSender.sender.wait -> sendInfo [order 3] : [sendACTSign == true]
      sendInfo -> SFSender.sender.transmission : {SFIndex = 3;
          | sendACTSign = false;}
      sendRandomSF -> SFSender.sender.transmission : {SFIndex = 1;
          | sendRandSFSign = false;}
      sendOK -> SFSender.sender.transmission : {SFIndex = 2;
          | sendOkSign = false;
          | init();
          | BA = true;
          | }
      SFSender.sender.transmission -> SFSender.sender : exit(SendHolder.hold)
          | {SDataOut = uint32(0);
          | SOutSign = false;
          | }
    state SendHolder [parallel]
      settings: executionOrder=2
      state end
      state hold
      note: 数据的发送需要持续42.7us
      end -> hold : enter(sender.transmission)
          | {
          | t1 = clock_Counter;
          | }
      (default) -> end
      hold -> end : [clock_Counter - t1 > 4.27]
  state MFSender [parallel]
    settings: executionOrder=2
    state sender [parallel]
      settings: executionOrder=1
      state sleep
      state wait
        entry:
        signal1 = true
      state transmission
        entry:
        signal1 = false;
        MDataOut = MFT(MFIndex);
        MOutSign = true;
        [acceptSF, acceptACT, acceptDomain] = setAcceptSignal(MDataOut);
      (default) -> sleep : {
          | init();
          | }
      sleep -> MFSender.sender.wait : [BA==true && clock_3M ~= clock_3M_shang]
          | {
          | clock_3M_shang = clock_3M;
          | }
      MFSender.sender.transmission -> sleep : exit(buffer.full)
          | {
          | MDataOut = uint32(0);
          | MOutSign = false;
          | MFIndex = MFIndex + 1;
          | }
      MFSender.sender.wait -> MFSender.sender.transmission : [trans1 == true]
    state buffer [parallel]
      settings: executionOrder=2
      note: 输出要保持42.7us
      state full
      state empty
      (default) -> empty
      full -> empty : [clock_Counter - t2 > 4.27]
      empty -> full : [enter(sender.transmission)]
          | {
          | t2 = clock_Counter;
          | }
  (default) -> MFSender
  data: f_code function_input; addr function_input; r function_output; addr function_input; r function_output; SFIndex local double; t1 local uint32; dataIn function_input uint32; SF function_output boolean; ACT function_output; Domain function_output; t2 local uint32; MFReceive input boolean; MDataOut output uint32; clock_3M data_store_memory; clock_Counter data_store_memory; MFIndex local; MFT local uint32 size=5; trans1 data_store_memory; signal1 data_store_memory; SFReceive input boolean; sendOkSign data_store_memory; sendRandSFSign data_store_memory; sendACTSign data_store_memory; SFT local uint32 size=3; SDataOut output uint32; MOutSign output boolean; SOutSign output boolean; isMaster local boolean; acceptSF data_store_memory; BA data_store_memory; clock_3M_shang local boolean; acceptACT data_store_memory; acceptDomain data_store_memory
  function r = getMF(f_code, addr):
    | function r = getMF(f_code, addr)
    | r = 3340042240;
    | r = r + bitshift(uint32(f_code), 12);
    | r = r + addr;
  function r = getSF(addr):
    | function r = getSF(addr)
    | r = 2833448960;
    | r = r + addr;
  function judgeMaster:
    | function judgeMaster
    | % 如果
    | if isMaster == true && SFIndex == 2
    |     isMaster = false;
    | end
  function [SF, ACT, Domain] = setAcceptSignal(dataIn):
    | function [SF, ACT, Domain] = setAcceptSignal(dataIn)
    | % 右移12位 仅保留帧头和fcode
    | dataInExAddr = bitshift(uint32(dataIn), -12);
    | % 先右移16位再左移4位 仅仅保留帧头
    | dataInStart = bitshift(bitshift(uint32(dataIn), -16), 4);
    | % 相减得到fcode
    | fcode = double(dataInExAddr - dataInStart);
    | SF = false;
    | Domain = false;
    | ACT = false;
    | if fcode == 0
    |     SF = true;
    | elseif fcode == 15
    |     ACT = true;
    | else
    |     Domain = true;
    | end
